simulink model "db4_2"  (R2018a)
settings: Solver=ode23  StartTime=0.0  StopTime=0.5  RelTol=1e-7  AbsTol=1e-9
values from neighbouring files (symbols this model uses):
  e = 0    [simulaciones.m]
  Iaref = str2num(get(findobj('Tag','variable1'),'String'))    [simulaciones.m]
  Kn = 0.6    [set_motor.m]
settings Model: ExtModeTrigMode=oneshot  ExtModeArmWhenConnect=off  Creator=Administrador  LastModifiedBy=Matias
settings SolverCC: AutoScaleAbsTol=off
settings DataIOCC: SaveFormat=Array  SignalLoggingSaveFormat=ModelDataLogs
settings OptimizationCC: BlockReduction=off  BooleanDataType=off  ExpressionDepthLimit=2147483647  InitFltsAndDblsToZero=on  LifeSpan=inf
settings DebuggingCC: SaveWithParameterizedLinksMsg=none  UnderspecifiedInitializationDetection=Classic  MergeDetectMultiDrivingBlocksExec=none  SignalResolutionControl=TryResolveAllWithWarning  MultiTaskDSMMsg=warning  MultiTaskCondExecSysMsg=none  FcnCallInpInsideContextMsg=warning  StateNameClashWarn=warning  SFUnexpectedBacktrackingDiag=warning  SFNoUnconditionalDefaultTransitionDiag=warning  SFExecutionAtInitializationDiag=none
settings HardwareCC: ProdBitPerPointer=32  ProdBitPerSizeT=32  ProdBitPerPtrDiffT=32  ProdLargestAtomicFloat=None  ProdIntDivRoundTo=Undefined  ProdEndianess=Unspecified  ProdWordSize=32  ProdHWDeviceType=32-bit Generic  TargetUnknown=on
settings ModelReferenceCC: PropagateSignalLabelsOutOfModel=off
settings RTWCC: TemplateMakefile=grt_vc.tmf
settings CodeAppCC: StateflowObjectComments=on
settings GRTTargetCC: TargetLangStandard=C89/C90 (ANSI)  CombineOutputUpdateFcns=off  GRTInterface=on
settings ConfigComp: CovMetricSettings=dw  CovHtmlReporting=on  CovSaveCumulativeToWorkspaceVar=on  CovSaveSingleToWorkspaceVar=on  CovExternalEMLEnable=off

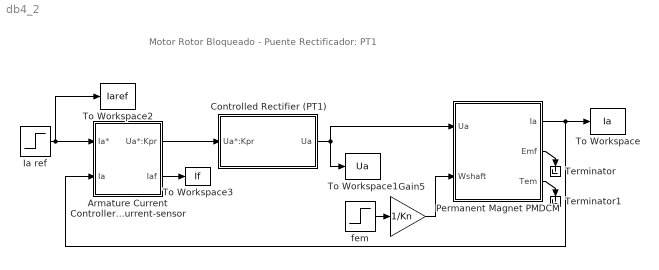
== system db4_2 ==
  note: Motor Rotor Bloqueado - Puente Rectificador: PT1
  Armature Current Controller (PI) with Current-sensor : Subsystem  mask(Armature Current Controller with Current-sensor){d=off, Kpi=0.0218, TIi=0.06, Kti=1, Tfi=0.008}
      mask prompts: d "Zero pre-compensation"; Kpi "Current Proportional Gain:"; TIi "Current Integral Gain:"; Kti "Current-sensor Proportional Gain:"; Tfi "Current-sensor Integral Gain:"
      mask init:
      | if d==1
      | TIi_c=TIi;
      | else
      | TIi_c=0;
      | end
  Controlled Rectifier (PT1) : Subsystem  mask(Controlled Rectifier (PT1)){Tpr=0.00167, Kpr=20}
      mask prompts: Tpr "Controlled Rectifier Integral Gain:"; Kpr "Controlled Rectifier Gain:"
      mask Display:
      | plot([0.45 0.8 0.8 0.45 0.45],[0.15 0.15 .85 .85 0.15])
      | plot(0.42+0.5*(0.1:0.02:0.7),0.2+0.3*log(1:0.2:7))
  Gain5 : Gain  Gain=1/Kn  SaturateOnIntegerOverflow=on  OutDataTypeStr=Inherit: Same as input  ParamDataTypeStr=Inherit: Same as input
  "Ia ref " : Step  Time=0  After=Iaref  SampleTime=0
  Permanent Magnet PMDCM : Subsystem  mask(Permanent Magnet PMDCM){La=0.003, Ra=0.05, k=6.7851, ic=0}
      mask prompts: La "Armature Inductance  [Hy]:"; Ra "Armature Resistance [Ohms]:"; k "Motor Constant:"; ic "Armature Current Initial Condition [Amp]:"
  Terminator : Terminator
  Terminator1 : Terminator
  To Workspace : ToWorkspace  VariableName=Ia  SampleTime=-1
  To Workspace1 : ToWorkspace  VariableName=Ua  SampleTime=-1
  To Workspace2 : ToWorkspace  VariableName=Iaref  SampleTime=-1
  To Workspace3 : ToWorkspace  VariableName=If  SampleTime=-1
  fem : Step  After=e  SampleTime=0
  wires:
  "Ia ref "/1 -> To Workspace2/1, Armature Current Controller (PI) with Current-sensor/1(Ia*)
  Armature Current Controller (PI) with Current-sensor/1(Ua*:Kpr) -> Controlled Rectifier (PT1)/1(Ua*:Kpr)
  Armature Current Controller (PI) with Current-sensor/2(Iaf) -> To Workspace3/1
  fem/1 -> Gain5/1
  Controlled Rectifier (PT1)/1(Ua) -> To Workspace1/1, Permanent Magnet PMDCM/1(Ua)
  Permanent Magnet PMDCM/1(Ia) -> To Workspace/1, Armature Current Controller (PI) with Current-sensor/2(Ia)
  Gain5/1 -> Permanent Magnet PMDCM/2(Wshaft)
  Permanent Magnet PMDCM/2(Emf) -> Terminator/1
  Permanent Magnet PMDCM/3(Tem) -> Terminator1/1

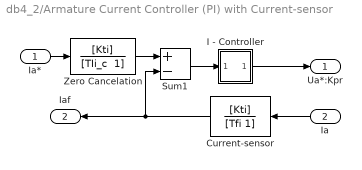
== system db4_2/Armature Current Controller (PI) with Current-sensor ==
  Ia* : Inport
  Ia : Inport  Port=2
  Current-sensor : TransferFcn  Numerator=[Kti]  Denominator=[Tfi 1]
  I - Controller : Subsystem  mask(PI Controller){P=Kpi, I=Kpi/TIi}
      mask prompts: P "Proportional:"; I "Integral:"
      mask help:
      | Enter expressions for proportional and  integral terms.
      | P+I/s
      mask Display: plot([0 0.001 5], [0 3 5])
  Sum1 : Sum  Inputs=+-  SaturateOnIntegerOverflow=on  InputSameDT=on  OutDataTypeStr=Inherit: Same as first input
  Zero Cancelation : TransferFcn  Numerator=[Kti]  Denominator="[TIi_c  1]"
  Ua*:Kpr : Outport
  Iaf : Outport  Port=2
  wires:
  Sum1/1 -> I - Controller/1(In_1)
  I - Controller/1(Out_1) -> Ua*:Kpr/1
  Ia/1 -> Current-sensor/1
  Current-sensor/1 -> Iaf/1, Sum1/2
  Zero Cancelation/1 -> Sum1/1
  Ia*/1 -> Zero Cancelation/1

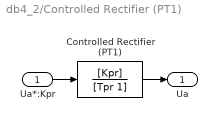
== system db4_2/Controlled Rectifier (PT1) ==
  Ua*:Kpr : Inport
  Controlled Rectifier (PT1) : TransferFcn  Numerator=[Kpr]  Denominator=[Tpr 1]
  Ua : Outport
  wires:
  Ua*:Kpr/1 -> Controlled Rectifier (PT1)/1
  Controlled Rectifier (PT1)/1 -> Ua/1

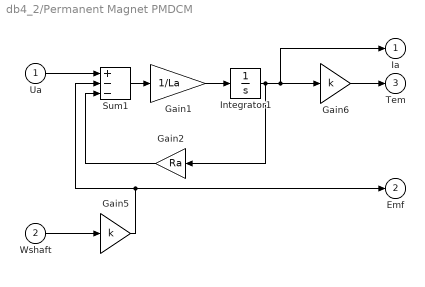
== system db4_2/Permanent Magnet PMDCM ==
  Ua : Inport
  Wshaft : Inport  Port=2
  Gain1 : Gain  Gain=1/La  SaturateOnIntegerOverflow=on  OutDataTypeStr=Inherit: Same as input  ParamDataTypeStr=Inherit: Same as input
  Gain2 : Gain  Gain=Ra  SaturateOnIntegerOverflow=on  OutDataTypeStr=Inherit: Same as input  ParamDataTypeStr=Inherit: Same as input
  Gain5 : Gain  Gain=k  SaturateOnIntegerOverflow=on  OutDataTypeStr=Inherit: Same as input  ParamDataTypeStr=Inherit: Same as input
  Gain6 : Gain  Gain=k  SaturateOnIntegerOverflow=on  OutDataTypeStr=Inherit: Same as input  ParamDataTypeStr=Inherit: Same as input
  Integrator1 : Integrator  InitialCondition=ic
  Sum1 : Sum  Inputs=+--  SaturateOnIntegerOverflow=on  InputSameDT=on  OutDataTypeStr=Inherit: Same as first input
  Ia : Outport
  Emf : Outport  Port=2
  Tem : Outport  Port=3
  wires:
  Wshaft/1 -> Gain5/1
  Gain5/1 -> Emf/1, Sum1/2
  Gain6/1 -> Tem/1
  Ua/1 -> Sum1/1
  Sum1/1 -> Gain1/1
  Gain1/1 -> Integrator1/1
  Gain2/1 -> Sum1/3
  Integrator1/1 -> Gain2/1, Ia/1, Gain6/1

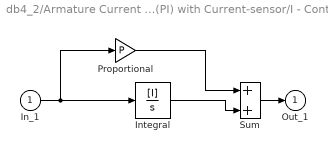
== system db4_2/Armature Current Controller (PI) with Current-sensor/I - Controller ==
  In_1 : Inport
  Integral : TransferFcn  Numerator=[I]  Denominator=[1 0]
  Proportional : Gain  Gain=P  SaturateOnIntegerOverflow=on  OutDataTypeStr=Inherit: Same as input  ParamDataTypeStr=Inherit: Same as input
  Sum : Sum  SaturateOnIntegerOverflow=on  InputSameDT=on  OutDataTypeStr=Inherit: Same as first input
  Out_1 : Outport
  wires:
  In_1/1 -> Proportional/1, Integral/1
  Sum/1 -> Out_1/1
  Integral/1 -> Sum/2
  Proportional/1 -> Sum/1
